simulink model "Control_TempHorno_simulink"  (R2017b)
settings: Solver=VariableStepAuto  StartTime=0.0  StopTime=50000  RelTol=1e-3
settings Model: Creator=diazm  LastModifiedBy=diazm

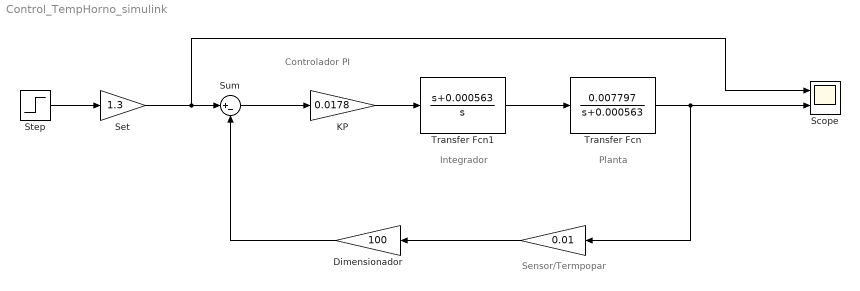
== system Control_TempHorno_simulink ==
  note: Controlador PI
  note: Planta
  note: Integrador
  note: Sensor/Termpopar
  " " : Gain  Gain=0.01
  "Dimensionador " : Gain  Gain=100
  KP : Gain  Gain=0.0178
  Scope : Scope  NumInputPorts=2
  Set : Gain  Gain=1.3
  Step : Step  SampleTime=0
  Sum : Sum  Inputs=|+-
  Transfer Fcn : TransferFcn  Numerator=[0.007797]  Denominator=[1 0.000563]
  Transfer Fcn1 : TransferFcn  Numerator=[1 0.000563]  Denominator=[1 0]
  wires:
  Sum/1 -> KP/1
  Step/1 -> Set/1
  KP/1 -> Transfer Fcn1/1
  Transfer Fcn1/1 -> Transfer Fcn/1
  Transfer Fcn/1 -> " "/1, Scope/2
  Set/1 -> Scope/1, Sum/1
  " "/1 -> "Dimensionador "/1
  "Dimensionador "/1 -> Sum/2
